simulink library "example_lib"  (Simulink 6.1)
libraries: xbsIndex_r4 x5, dsparch4 x1, dspobslib x1, example_lib x1
settings Model: Creator=singhj  LastModifiedBy=singhj

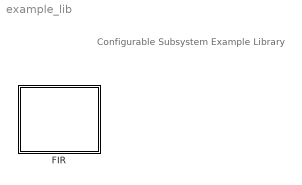
== system example_lib ==
  note: Configurable Subsystem
      | Example Library
  FIR : Subsystem  mask{coef=[0 0], latency=4}
      mask prompts: coef "Coefficients"
      mask help:
      | This masked subsystem is used simply to setup some workspace variables with defualt values that are used by the configurable subsystem block choices below it.
      |
      | This mask is useful only for manipulating the blocks within the library. It does nothing for copies of the configurable subsystem that are used in Simulink models. The template block underneath this level of hierarchy has the actual mask that will be presented to the designer when the block is added to a model.
      mask Display: disp('FIR LIB');

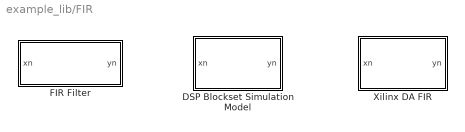
== system example_lib/FIR ==
  DSP Blockset Simulation Model : Subsystem
  FIR Filter : Subsystem  BlockChoice=DSP Blockset Simulation Model  mask{coef=fir1(16,0.5), latency=3}
      mask prompts: coef "Filter Coefficient Vector"
      settings: TemplateBlock=self  MemberBlocks=DSP Blockset Simulation Model,Xilinx DA FIR
  Xilinx DA FIR : Subsystem

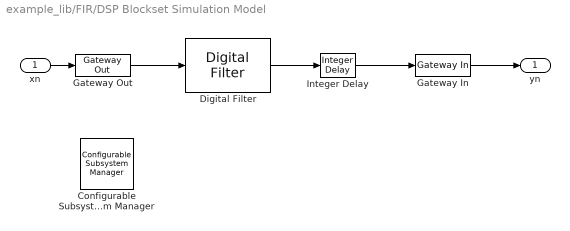
== system example_lib/FIR/DSP Blockset Simulation Model ==
  xn : Inport  Port=1  LatchInput=off
  Configurable Subsystem Manager : xbsIndex_r4/Configurable Subsystem Manager  Tag=xcfgMgr  block_type=configsubsys
      settings: AttributesFormatString=Configurable Subsystem\nManager
  Digital Filter : dsparch4/Digital Filter  DialogController=dspDDGCreate  DialogControllerArgs=DataTag0  TypePopup=FIR (all zeros)  IIRFiltStruct=Direct form II transposed  AllPoleFiltStruct=Direct form  FIRFiltStruct=Direct form  CoeffSource=Specify via dialog  NumCoeffs=coef  DenCoeffs=[1 0.1]  BiQuadCoeffs=[1 0.3 0.4 1 0.1 0.2]  LatticeCoeffs=[0.2 0.4]  denIgnore=on  FiltPerSampPopup=One filter per frame  IC=0  ICnum=0  ICden=0  roundingMode=Floor  overflowMode=off  ScaleValues=1  scaleValueFracLength=14  stageInFracLength=15  stageOutFracLength=15
  Gateway In : xbsIndex_r4/Gateway In  arith_type="Signed  (2's comp)"  n_bits=21  bin_pt=17  period=1  dbl_ovrd=off  timing_constraint=None  locs_specified=off  LOCs={}  block_type=gatewayin
      settings: infoedit="Gateway in block.  Converts inputs of type Simulink integer, double and fixed point to  Xilinx fixed point type.<P><P>Hardware notes:  In hardware these blocks become top level input ports."  xl_area=[0, 0, 0, 0, 0, 0, 0]  block_version=VER_STRING_GOES_HERE
  Gateway Out : xbsIndex_r4/Gateway Out  hdl_port=on  timing_constraint=None  locs_specified=off  LOCs={}  block_type=gatewayout
      settings: infoedit="Gateway out block.  Converts Xilinx fixed point inputs into ouputs of type Simulink integer, double, or fixed point.<P><P>Hardware notes:  In hardware these blocks become top level output ports or are discarded, depending on how they are configured."  xl_area=[0, 0, 0, 0, 0, 0, 0]  block_version=VER_STRING_GOES_HERE
  Integer Delay : dspobslib/Integer Delay  delay=latency  ic=0  reset_popup=None
  yn : Outport
  wires:
  xn/1 -> Gateway Out/1
  Gateway In/1 -> yn/1
  Digital Filter/1 -> Integer Delay/1
  Integer Delay/1 -> Gateway In/1
  Gateway Out/1 -> Digital Filter/1

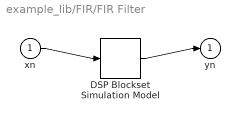
== system example_lib/FIR/FIR Filter ==
  xn : Inport  Port=1  LatchInput=off
  DSP Blockset Simulation Model : example_lib/FIR/DSP Blockset Simulation Model
  yn : Outport
  wires:
  xn/1 -> DSP Blockset Simulation Model/1
  DSP Blockset Simulation Model/1 -> yn/1

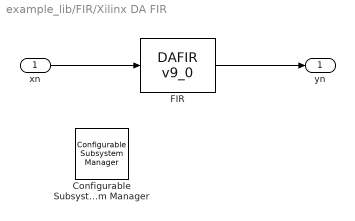
== system example_lib/FIR/Xilinx DA FIR ==
  xn : Inport  Port=1  LatchInput=off
  Configurable Subsystem Manager : xbsIndex_r4/Configurable Subsystem Manager  Tag=xcfgMgr  block_type=configsubsys
      settings: AttributesFormatString=Configurable Subsystem\nManager
  FIR : xbsIndex_r4/DAFIR v9_0   coef=coef  structure=Inferred from Coefficients  coef_arith_type="Signed  (2's complement)"  coef_n_bits=12  coef_bin_pt=11  over_sample=1  reload=off  valids=off  latency=latency  num_channels=1  serial_input=off  polyphase_behavior="Single Rate:  sample in - sample out"  dbl_ovrd=off  explicit_period=off  period=1  block_type=fir
      settings: infoedit="Hardware notes: Implemented using distributed arithmetic (DA).  The hardware over sampling rate determines the degree of parallelism.  A rate of one produces a fully parallel DA filter.  A rate of n (resp., n+1) for an n-bit input signal produces a fully serial implementation for a non-symmetric (resp., symmetric) impulse response.  Intermediate values produce implementations with intermediate levels of parallelism."  xl_area=[0, 0, 0, 0, 0, 0, 0]  block_version=VER_STRING_GOES_HERE
  yn : Outport
  wires:
  FIR/1 -> yn/1
  xn/1 -> FIR/1
